simulink model "Function1_2018a"  (R2018a)
settings: Solver=FixedStepDiscrete  StartTime=0.0  StopTime=0.1  FixedStep=0.1  RelTol=1e-3  EnableMultiTasking=on
settings Model: Creator=bzhan  LastModifiedBy=bzhan
settings SolverCC: AutoInsertRateTranBlk=on
settings DataIOCC: LimitDataPoints=on  ReturnWorkspaceOutputs=on
settings OptimizationCC: LifeSpan=inf
settings DebuggingCC: AllowSymbolicDim=off  SFUnexpectedBacktrackingDiag=warning  SFNoUnconditionalDefaultTransitionDiag=warning  SFExecutionAtInitializationDiag=none
settings CodeAppCC: StateflowObjectComments=on
settings GRTTargetCC: TargetLangStandard=C89/C90 (ANSI)
settings ConfigComp: CovMetricSettings=dw  CovHtmlReporting=on  CovSaveCumulativeToWorkspaceVar=on  CovSaveSingleToWorkspaceVar=on  CovShowResultsExplorer=off  CovExternalEMLEnable=off  CovSFcnEnable=off

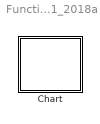
== system Function1_2018a ==
  Chart : Stateflow chart  TreatAsAtomicUnit=on

== stateflow chart Function1_2018a/Chart ==
  state A
    en: f("en_A")
  state B
    en: f("en_B")
  (default) -> A
  A -> B : [compute(3)==15]
  data: x function_input; y function_output; s function_input
  function y = compute(x):
    | function y = compute(x)
    |   y = x + 1;
    |   z = y * y;
    |   y = z - 1;
  function f(s):
    | function f(s)
    |   fprintf(s+"\n");
